simulink model "ex46improver"  (R2025b)
settings: Solver=VariableStepAuto  StartTime=0.0  StopTime=250  RelTol=1e-3
values from neighbouring files (symbols this model uses):
  K = nmpc_design_st2(par)    [ex16.m]    (also in ex26.m; ex46.m)
  ref = [6971 0 0 0 0]    [ex16.m]    (also in ex26.m = [9192.3, 0.22, 0.026, 0, 0]; ex46.m = [0;0])
settings Model: Creator=Esteban  LastModifiedBy=Esteban

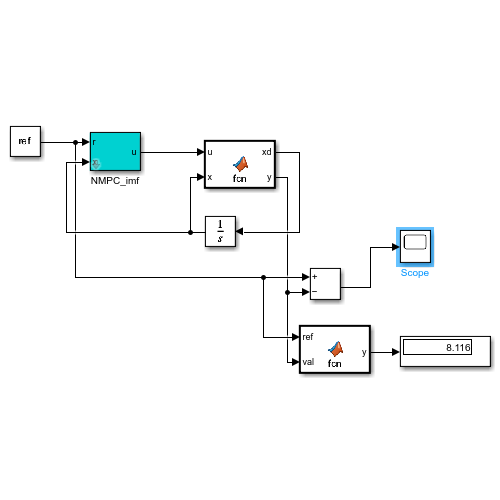
[thumbnail: Simulink's stored preview of the top-level diagram]
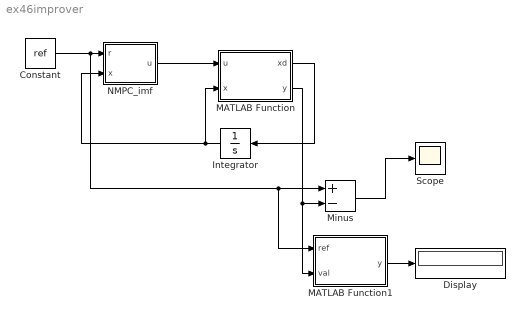
== system ex46improver ==
  Constant : Constant  Value=ref
  Display : Display
  Integrator : Integrator  InitialCondition=[-3000;600;0]
  MATLAB Function : MATLAB Function  TreatAsAtomicUnit=on
  MATLAB Function1 : MATLAB Function  TreatAsAtomicUnit=on
  Minus : Sum  Inputs=+-
  NMPC_imf : Subsystem  mask{K=K}
      mask prompts: K "NMPC structure"
  Scope : Scope
      settings: ActiveDisplayYMinimum=-1347.6652130875234  ActiveDisplayYMaximum=1698.1119160415669
  wires:
  Constant/1 -> Minus/1, MATLAB Function1/1(ref), NMPC_imf/1(r)
  NMPC_imf/1(u) -> MATLAB Function/1(u)
  MATLAB Function/1(xd) -> Integrator/1
  Integrator/1 -> NMPC_imf/2(x), MATLAB Function/2(x)
  Minus/1 -> Scope/1
  MATLAB Function/2(y) -> MATLAB Function1/2(val), Minus/2
  MATLAB Function1/1(y) -> Display/1

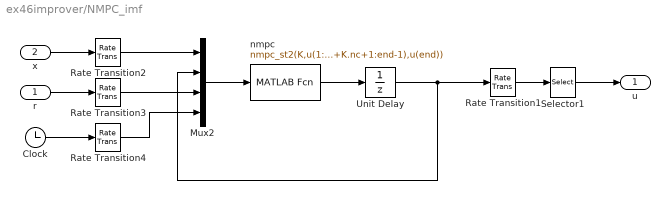
== system ex46improver/NMPC_imf ==
  r : Inport
  x : Inport  Port=2
  Clock : Clock
  Mux2 : Mux
  Rate Transition{1..4} (4 alike) : RateTransition  OutPortSampleTime=K.Ts
  Selector1 : Selector  InputPortWidth=K.nc  IndexOptions=Index vector (dialog)  Indices=1:K.nu  OutputSizes=1
  Unit Delay : UnitDelay  InitialCondition=zeros(K.nc,1)  SampleTime=K.Ts  HasFrameUpgradeWarning=on
  nmpc : MATLABFcn  MATLABFcn=nmpc_st2(K,u(1:K.nx),u(K.nx+1:K.nx+K.nc),u(K.nx+K.nc+1:end-1),u(end))  OutputDimensions=K.nc
  u : Outport  PortDimensions=K.nu
  wires:
  x/1 -> Rate Transition2/1
  Unit Delay/1 -> Rate Transition1/1, Mux2/2
  Mux2/1 -> nmpc/1
  r/1 -> Rate Transition3/1
  Rate Transition2/1 -> Mux2/1
  Rate Transition1/1 -> Selector1/1
  Rate Transition3/1 -> Mux2/3
  nmpc/1 -> Unit Delay/1
  Selector1/1 -> u/1
  Clock/1 -> Rate Transition4/1
  Rate Transition4/1 -> Mux2/4

== matlab function ex46improver/MATLAB Function ==
  data: xd output; u input; y output; x input
function [xd,y] = fcn(u,x)
th = x(3,:);
l = 1.5;
xd = [u(1)*cos(th);
      u(1)*sin(th);
      u(1)/l*tan(u(2))];

y = [x(1);x(2)];

== matlab function ex46improver/MATLAB Function1 ==
  data: ref input; y output; val input
function y = fcn(ref,val)

y = norm(ref-val);
